simulink model "pitch_attitude_hold_autopilot_2018"  (R2020a)
settings: Solver=VariableStepAuto  StartTime=0.0  StopTime=50  RelTol=1e-3
libraries: simulink x1
settings Model: Creator=parth  LastModifiedBy=parth
settings DebuggingCC: ArithmeticOperatorsInVariantConditions=warning
settings SFSimCC: CustomCodeUndefinedFunction=UseInterfaceOnly

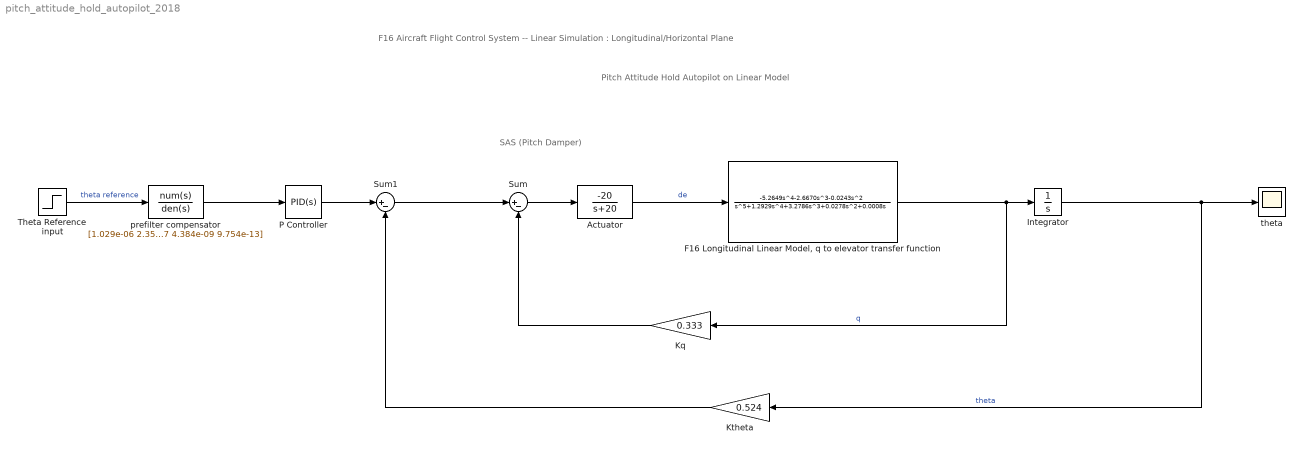
== system pitch_attitude_hold_autopilot_2018 ==
  note: SAS (Pitch Damper)
  note: F16 Aircraft Flight Control System -- Linear Simulation : Longitudinal/Horizontal Plane
  note: Pitch Attitude Hold Autopilot on Linear Model
  Actuator : TransferFcn  Numerator=[-20]  Denominator=[1, 20]
  "F16 Longitudinal Linear Model, q to elevator transfer function" : TransferFcn  Numerator="[0   -5.2649   -2.6670   -0.0243   -0.0000 0.000]"  Denominator="[1.0000    1.2929    3.2786    0.0278    0.0008 0.000]"
  Integrator : Integrator
  Kq : Gain  Gain=0.333
  Ktheta : Gain  Gain=0.524
  P Controller : simulink/Continuous/PID Controller  Controller=PID  Form=Parallel  TimeDomain=Continuous-time  UseExternalTs=off  SampleTime=-1  IntegratorMethod=Forward Euler  FilterMethod=Forward Euler  ControllerParametersSource=internal  P=1.092  I=0  D=0  UseFilter=on  N=100  TunerSelectOption=Transfer Function Based (PID Tuner App)  InitialConditionSource=internal  InitialConditionForIntegrator=0  InitialConditionForFilter=0  DifferentiatorICPrevScaledInput=0  ExternalReset=none  TrackingMode=off  Kt=1  LimitOutput=off  UpperSaturationLimit=inf  LowerSaturationLimit=-inf  LinearizeAsGain=on  AntiWindupMode=none  Kb=1  POutMin=[]  POutMax=[]  IOutMin=[]  IOutMax=[]  DOutMin=[]  DOutMax=[]  NOutMin=[]  NOutMax=[]  SumOutMin=[]  SumOutMax=[]  SaturationOutMin=[]  SaturationOutMax=[]  PParamMin=[]  PParamMax=[]  IParamMin=[]  IParamMax=[]  DParamMin=[]  DParamMax=[]  NParamMin=[]  NParamMax=[]  KbParamMin=[]  KbParamMax=[]  KtParamMin=[]  KtParamMax=[]  KbOutMin=[]  KbOutMax=[]  KtOutMin=[]  KtOutMax=[]  IntegratorOutMin=[]  IntegratorOutMax=[]  FilterOutMin=[]  FilterOutMax=[]  SumI1OutMin=[]  SumI1OutMax=[]  SumI2OutMin=[]  SumI2OutMax=[]  SumI3OutMin=[]  SumI3OutMax=[]  SumI4OutMin=[]  SumI4OutMax=[]  SumDOutMin=[]  SumDOutMax=[]  DifferentiatorOutMin=[]  DifferentiatorOutMax=[]  FilterDiffOutCoefMin=[]  FilterDiffOutCoefMax=[]  ReciprocalOutMin=[]  ReciprocalOutMax=[]  SumDenOutMin=[]  SumDenOutMax=[]  SumNumOutMin=[]  SumNumOutMax=[]  DivideOutMin=[]  DivideOutMax=[]  UdiffTsProdOutMin=[]  UdiffTsProdOutMax=[]  NTsProdOutMin=[]  NTsProdOutMax=[]  UintegralTsProdOutMin=[]  UintegralTsProdOutMax=[]  UngainTsProdOutMin=[]  UngainTsProdOutMax=[]  IntegratorContinuousStateAttributes=''  IntegratorStateMustResolveToSignalObject=off  IntegratorRTWStateStorageClass=Auto  FilterContinuousStateAttributes=''  FilterStateMustResolveToSignalObject=off  FilterRTWStateStorageClass=Auto  ParallelPVariant=InternalParameters  IdealPVariant=Disabled  IVariant=InternalParameters  DVariant=InternalParameters  IntegratorVariant=Continuous  SatVariant=Disabled  AWVariant=Passthrough  PCopyVariant=Disabled  TRVariant=Disabled  FdbkBlocksVariant=Forward  IdealPFdbkVariant=Disabled  SatFdbkVariant=Disabled  DerivativeFilterVariant=ContFilter  NVariant=InternalParameters  NCopyVariant=Disabled  FilterICVariant=InternalICsFilter  IntegratorICVariant=InternalICs  ExternalResetVariant=Disabled  TRSumVariant=Passthrough  SumFdbkVariant=Disabled  SumVariant=Sum_PID  TsampFilterVariant=InternalTs  TsampNgainVariant=Passthrough  TsampIntegralVariant=Passthrough
  Sum : Sum  Inputs=|+-
  Sum1 : Sum  Inputs=|+-
  Theta Reference input : Step  Time=0  SampleTime=0
  prefilter compensator : TransferFcn  Numerator=[1.029e-06 2.35e-07 2.227e-09 9.754e-13]  Denominator=[9.482e-07 4.803e-07 4.384e-09 9.754e-13]
  theta : Scope
  wires:
  Theta Reference input/1 -> prefilter compensator/1  "theta reference"
  prefilter compensator/1 -> P Controller/1
  Ktheta/1 -> Sum1/2
  P Controller/1 -> Sum1/1
  Sum1/1 -> Sum/1
  Actuator/1 -> "F16 Longitudinal Linear Model, q to elevator transfer function"/1  "de"
  Sum/1 -> Actuator/1
  "F16 Longitudinal Linear Model, q to elevator transfer function"/1 -> Kq/1, Integrator/1  "q"
  Integrator/1 -> Ktheta/1, theta/1  "theta"
  Kq/1 -> Sum/2
